simulink model "SF107A_MotRplCoggCmd"  (R2013b)
settings: Solver=FixedStepDiscrete  SolverMode=SingleTasking  StartTime=0.0  StopTime=1  FixedStep=0.002  RelTol=1e-3
undefined symbols (not defined in the file): ARCHGLBPRM_2PI_ULS_F32, ININITRNIDXCON_CNT_U16, ITRNIDXCON_CNT_U08, MotRplCoggCmdHrmncOrder1Elec, MotRplCoggCmdHrmncOrder2Elec, MotRplCoggCmdHrmncOrder3Elec, NvmGetErrSts1, ONEOVER12_MOTREV_F32, ONEOVER2PI_ULS_F32
libraries: NxtrNvM x3, NxtrLim x3, NxtrMath x3, simulink x2, FloatToFixd x2, FixdToFloat x2
(part 2 of 2)

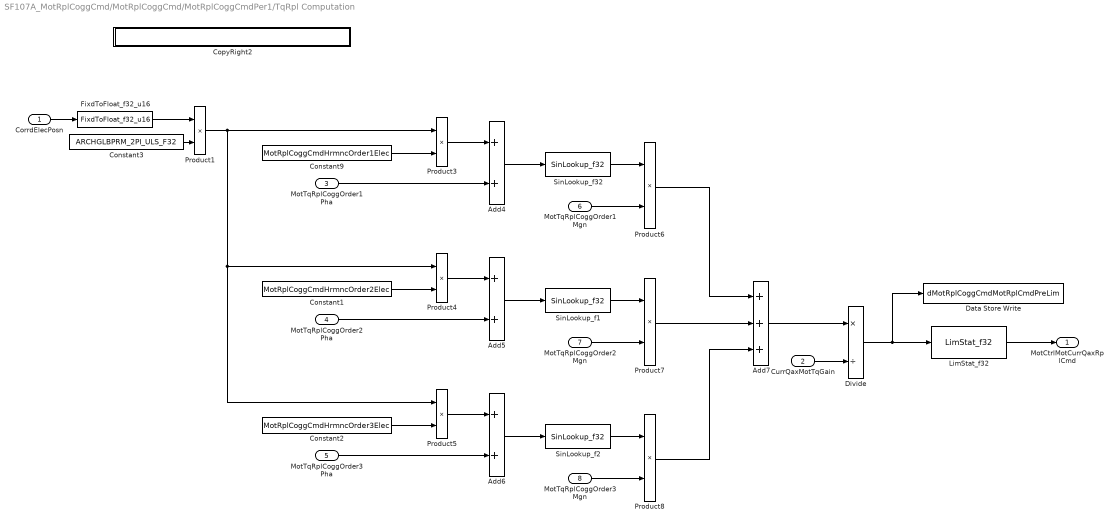
== system SF107A_MotRplCoggCmd/MotRplCoggCmd/MotRplCoggCmdPer1/TqRpl Computation ==
  CorrdElecPosn : Inport
  CurrQaxMotTqGain : Inport  Port=2
  MotTqRplCoggOrder1Pha : Inport  Port=3
  MotTqRplCoggOrder2Pha : Inport  Port=4
  MotTqRplCoggOrder3Pha : Inport  Port=5
  MotTqRplCoggOrder1Mgn : Inport  Port=6
  MotTqRplCoggOrder2Mgn : Inport  Port=7
  MotTqRplCoggOrder3Mgn : Inport  Port=8
  Add4 : Sum  RequirementInfo="{'linktype_rmi_doors' '0000bb46 (/E-STEER Core/SubSystem Specifications/Application Functions/SF99/SF107A Cogging and Ripple Command Generation)' '#SF107A_55' 'true' 'REQ:  SF107A_55' '' } %GIDa_98f659b8_5f56_4abb_a016_23e4f1dc427c"
  Add5 : Sum  RequirementInfo="{'linktype_rmi_doors' '0000bb46 (/E-STEER Core/SubSystem Specifications/Application Functions/SF99/SF107A Cogging and Ripple Command Generation)' '#SF107A_55' 'true' 'REQ:  SF107A_55' '' } %GIDa_a031d6e0_d51d_47e6_9a68_2e9a42cf15d5"
  Add6 : Sum  RequirementInfo="{'linktype_rmi_doors' '0000bb46 (/E-STEER Core/SubSystem Specifications/Application Functions/SF99/SF107A Cogging and Ripple Command Generation)' '#SF107A_55' 'true' 'REQ:  SF107A_55' '' } %GIDa_8917c88f_1d70_4c7d_a0e1_dd355f06626f"
  Add7 : Sum  RequirementInfo="{'linktype_rmi_doors' '0000bb46 (/E-STEER Core/SubSystem Specifications/Application Functions/SF99/SF107A Cogging and Ripple Command Generation)' '#SF107A_54' 'true' 'REQ:  SF107A_54' '' } %GIDa_e539927c_b2fd_444b_9336_b367779ce02b"  Inputs=+++
  Constant1 : Constant  RequirementInfo="{'linktype_rmi_doors' '0000bb46 (/E-STEER Core/SubSystem Specifications/Application Functions/SF99/SF107A Cogging and Ripple Command Generation)' '#SF107A_57' 'true' 'REQ:  SF107A_57' '' } %GIDa_f072efd8_bbd4_4d38_ae65_803309e61bdb"  Value=MotRplCoggCmdHrmncOrder2Elec
  Constant2 : Constant  RequirementInfo="{'linktype_rmi_doors' '0000bb46 (/E-STEER Core/SubSystem Specifications/Application Functions/SF99/SF107A Cogging and Ripple Command Generation)' '#SF107A_57' 'true' 'REQ:  SF107A_57' '' } %GIDa_2383bf9d_24cd_4efb_88f1_9d3d7a1f1b92"  Value=MotRplCoggCmdHrmncOrder3Elec
  Constant3 : Constant  Value=ARCHGLBPRM_2PI_ULS_F32
  Constant9 : Constant  RequirementInfo="{'linktype_rmi_doors' '0000bb46 (/E-STEER Core/SubSystem Specifications/Application Functions/SF99/SF107A Cogging and Ripple Command Generation)' '#SF107A_57' 'true' 'REQ:  SF107A_57' '' } %GIDa_68103fb0_c239_4eaa_ade4_33adb71360ab"  Value=MotRplCoggCmdHrmncOrder1Elec
  CopyRight2 : Subsystem  Description=|  mask(Copyright Information){none=on}
      | Copyright info block.                                               
      |                                                                     
      | Place copyright information at the top of every subsystem in design.
      mask prompts: none "No parameters"
      mask help: Place copyright information at the top of every subsystem in design.
      mask Display:
      | NxtrConf = 'Nexteer Confidential';
      | 
      | sys = bdroot; %handle for the current model ("system")
      | first = get_param(sys,'Created');
      | if(isempty(first))
      |     first = datestr(now,'yyyy');
      | else
      |     first = first(end-3:end);  %year is last four digits
      | end
      | 
      | last = get_param(sys,'LastModifiedDate');
      | if isempty(last)
      |     last = datestr(now,'yyyy');
      | else
      |     last = last(end-3:end);
      | end
      | 
      | if strcmp(first,last)
      |     fprintf('%s -- Copyright %s Nexteer',NxtrConf,first)
      | else
      |     fprintf('%s -- %s%s- %s Nexteer',NxtrConf,char(169),first,last)
      | end
  Data Store Write : DataStoreWrite  DataStoreName=dMotRplCoggCmdMotRplCmdPreLim
  Divide : Product  RequirementInfo="{'linktype_rmi_doors' '0000bb46 (/E-STEER Core/SubSystem Specifications/Application Functions/SF99/SF107A Cogging and Ripple Command Generation)' '#SF107A_53' 'true' 'REQ:  SF107A_53' '' } %GIDa_313ededd_ac17_4f1e_9f46_14b7bb626f21"  Inputs=*/
  FixdToFloat_f32_u16 : FixdToFloat/FixdToFloat_f32_u16  Param1=16
  LimStat_f32 : NxtrLim/LimStat_f32  LoLim=MOTRPLCMDLOLIM_AMPR_F32  HiLim=MOTRPLCMDHILIM_AMPR_F32
      settings: AttributesFormatString=|
      | Low Limit: %<LoLim>
      | High Limit:%<HiLim>
  Product1 : Product  RequirementInfo="{'linktype_rmi_doors' '0000bb46 (/E-STEER Core/SubSystem Specifications/Application Functions/SF99/SF107A Cogging and Ripple Command Generation)' '#SF107A_55' 'true' 'REQ:  SF107A_55' '' } %GIDa_600ef9ea_cc95_47b9_9c04_0003a85331d8"
  Product3 : Product  RequirementInfo="{'linktype_rmi_doors' '0000bb46 (/E-STEER Core/SubSystem Specifications/Application Functions/SF99/SF107A Cogging and Ripple Command Generation)' '#SF107A_55' 'true' 'REQ:  SF107A_55' '' } %GIDa_3469ba64_b899_493e_9d33_70a47609b0d9"
  Product4 : Product  RequirementInfo="{'linktype_rmi_doors' '0000bb46 (/E-STEER Core/SubSystem Specifications/Application Functions/SF99/SF107A Cogging and Ripple Command Generation)' '#SF107A_55' 'true' 'REQ:  SF107A_55' '' } %GIDa_836095c6_cb2f_45b0_8f00_b099e6d0c57b"
  Product5 : Product  RequirementInfo="{'linktype_rmi_doors' '0000bb46 (/E-STEER Core/SubSystem Specifications/Application Functions/SF99/SF107A Cogging and Ripple Command Generation)' '#SF107A_55' 'true' 'REQ:  SF107A_55' '' } %GIDa_688eee67_c46e_432a_b632_56124a9b3371"
  Product6 : Product  RequirementInfo="{'linktype_rmi_doors' '0000bb46 (/E-STEER Core/SubSystem Specifications/Application Functions/SF99/SF107A Cogging and Ripple Command Generation)' '#SF107A_55' 'true' 'REQ:  SF107A_55' '' } %GIDa_9339410d_3093_41b9_852e_c1514004436d"
  Product7 : Product  RequirementInfo="{'linktype_rmi_doors' '0000bb46 (/E-STEER Core/SubSystem Specifications/Application Functions/SF99/SF107A Cogging and Ripple Command Generation)' '#SF107A_55' 'true' 'REQ:  SF107A_55' '' } %GIDa_a170c4db_a53c_4e52_92bc_536d39694cf5"
  Product8 : Product  RequirementInfo="{'linktype_rmi_doors' '0000bb46 (/E-STEER Core/SubSystem Specifications/Application Functions/SF99/SF107A Cogging and Ripple Command Generation)' '#SF107A_55' 'true' 'REQ:  SF107A_55' '' } %GIDa_e07e829d_dd69_4b61_917b_3f5e8f99ba6e"
  SinLookup_f1 : NxtrMath/SinLookup_f32  RequirementInfo="{'linktype_rmi_doors' '0000bb46 (/E-STEER Core/SubSystem Specifications/Application Functions/SF99/SF107A Cogging and Ripple Command Generation)' '#SF107A_55' 'true' 'REQ:  SF107A_55' '' } %GIDa_3d2458f1_7193_4548_807d_b5b7c1c38197"
  SinLookup_f2 : NxtrMath/SinLookup_f32  RequirementInfo="{'linktype_rmi_doors' '0000bb46 (/E-STEER Core/SubSystem Specifications/Application Functions/SF99/SF107A Cogging and Ripple Command Generation)' '#SF107A_55' 'true' 'REQ:  SF107A_55' '' } %GIDa_b6162dde_f64c_4e1b_975d_22547d97ab53"
  SinLookup_f32 : NxtrMath/SinLookup_f32  RequirementInfo="{'linktype_rmi_doors' '0000bb46 (/E-STEER Core/SubSystem Specifications/Application Functions/SF99/SF107A Cogging and Ripple Command Generation)' '#SF107A_55' 'true' 'REQ:  SF107A_55' '' } %GIDa_5133dd47_8220_4bd1_8174_beaea066f0ab"
  MotCtrlMotCurrQaxRplCmd : Outport
  wires:
  Add6/1 -> SinLookup_f2/1
  Product4/1 -> Add5/1
  Product6/1 -> Add7/1
  MotTqRplCoggOrder3Mgn/1 -> Product8/2
  Constant1/1 -> Product4/2
  Product3/1 -> Add4/1
  Add4/1 -> SinLookup_f32/1
  MotTqRplCoggOrder2Mgn/1 -> Product7/2
  MotTqRplCoggOrder3Pha/1 -> Add6/2
  SinLookup_f1/1 -> Product7/1
  Add7/1 -> Divide/1
  Product8/1 -> Add7/3
  CorrdElecPosn/1 -> FixdToFloat_f32_u16/1
  Product5/1 -> Add6/1
  MotTqRplCoggOrder2Pha/1 -> Add5/2
  Constant2/1 -> Product5/2
  SinLookup_f32/1 -> Product6/1
  Product7/1 -> Add7/2
  Add5/1 -> SinLookup_f1/1
  Divide/1 -> LimStat_f32/1, Data Store Write/1
  CurrQaxMotTqGain/1 -> Divide/2
  Constant9/1 -> Product3/2
  SinLookup_f2/1 -> Product8/1
  MotTqRplCoggOrder1Pha/1 -> Add4/2
  MotTqRplCoggOrder1Mgn/1 -> Product6/2
  LimStat_f32/1 -> MotCtrlMotCurrQaxRplCmd/1
  Product1/1 -> Product4/1, Product5/1, Product3/1
  FixdToFloat_f32_u16/1 -> Product1/1
  Constant3/1 -> Product1/2

== system SF107A_MotRplCoggCmd/MotRplCoggCmd/SetMotCoggCmdPrm/CopyRight1 ==

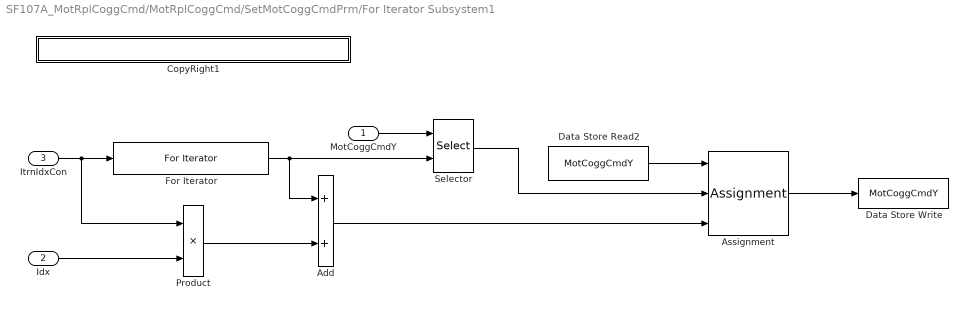
== system SF107A_MotRplCoggCmd/MotRplCoggCmd/SetMotCoggCmdPrm/For Iterator Subsystem1 ==
  MotCoggCmdY : Inport
  Idx : Inport  Port=2
  ItrnIdxCon : Inport  Port=3
  Add : Sum
  Assignment : Assignment  IndexMode=Zero-based  IndexOptions=Index vector (port)  Indices=1  OutputSizes=128
  CopyRight1 : Subsystem  Description=|  mask(Copyright Information){none=on}
      | Copyright info block.                                               
      |                                                                     
      | Place copyright information at the top of every subsystem in design.
      mask prompts: none "No parameters"
      mask help: Place copyright information at the top of every subsystem in design.
      mask Display:
      | NxtrConf = 'Nexteer Confidential';
      | 
      | sys = bdroot; %handle for the current model ("system")
      | first = get_param(sys,'Created');
      | if(isempty(first))
      |     first = datestr(now,'yyyy');
      | else
      |     first = first(end-3:end);  %year is last four digits
      | end
      | 
      | last = get_param(sys,'LastModifiedDate');
      | if isempty(last)
      |     last = datestr(now,'yyyy');
      | else
      |     last = last(end-3:end);
      | end
      | 
      | if strcmp(first,last)
      |     fprintf('%s -- Copyright %s Nexteer',NxtrConf,first)
      | else
      |     fprintf('%s -- %s%s- %s Nexteer',NxtrConf,char(169),first,last)
      | end
  Data Store Read2 : DataStoreRead  DataStoreName=MotCoggCmdY
  Data Store Write : DataStoreWrite  DataStoreName=MotCoggCmdY
  For Iterator : ForIterator  IterationSource=external  IterationLimit=127  IndexMode=Zero-based  IterationVariableDataType=int16
  Product : Product  OutDataTypeStr=int16
  Selector : Selector  IndexMode=Zero-based  InputPortWidth=128  IndexOptions=Index vector (port)  Indices=[1 3]  OutputSizes=1
  wires:
  Data Store Read2/1 -> Assignment/1
  Product/1 -> Add/2
  MotCoggCmdY/1 -> Selector/1
  Assignment/1 -> Data Store Write/1
  For Iterator/1 -> Add/1, Selector/2
  Idx/1 -> Product/2
  ItrnIdxCon/1 -> Product/1, For Iterator/1
  Add/1 -> Assignment/3
  Selector/1 -> Assignment/2

== system SF107A_MotRplCoggCmd/MotRplCoggCmd/GetMotCoggCmdPrm/For Iterator Subsystem/CopyRight1 ==

== system SF107A_MotRplCoggCmd/MotRplCoggCmd/MotRplCoggCmdInit1/NVM is NOT okay/CopyRight2 ==

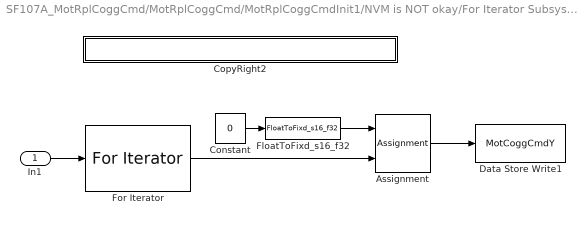
== system SF107A_MotRplCoggCmd/MotRplCoggCmd/MotRplCoggCmdInit1/NVM is NOT okay/For Iterator Subsystem ==
  In1 : Inport
  Assignment : Assignment  IndexMode=Zero-based  OutputInitialize=Specify size for each dimension in table  IndexOptions=Index vector (port)  Indices=1  OutputSizes=512
  Constant : Constant  Value=0  OutDataTypeStr=single
      settings: AttributesFormatString=%<OutDataTypeStr>
  CopyRight2 : Subsystem  Description=|  mask(Copyright Information){none=on}
      | Copyright info block.                                               
      |                                                                     
      | Place copyright information at the top of every subsystem in design.
      mask prompts: none "No parameters"
      mask help: Place copyright information at the top of every subsystem in design.
      mask Display:
      | NxtrConf = 'Nexteer Confidential';
      | 
      | sys = bdroot; %handle for the current model ("system")
      | first = get_param(sys,'Created');
      | if(isempty(first))
      |     first = datestr(now,'yyyy');
      | else
      |     first = first(end-3:end);  %year is last four digits
      | end
      | 
      | last = get_param(sys,'LastModifiedDate');
      | if isempty(last)
      |     last = datestr(now,'yyyy');
      | else
      |     last = last(end-3:end);
      | end
      | 
      | if strcmp(first,last)
      |     fprintf('%s -- Copyright %s Nexteer',NxtrConf,first)
      | else
      |     fprintf('%s -- %s%s- %s Nexteer',NxtrConf,char(169),first,last)
      | end
  Data Store Write1 : DataStoreWrite  DataStoreName=MotCoggCmdY
  FloatToFixd_s16_f32 : FloatToFixd/FloatToFixd_s16_f32  Param1=14
  For Iterator : ForIterator  IterationSource=external  IterationLimit=512  IndexMode=Zero-based  IterationVariableDataType=int16
  wires:
  In1/1 -> For Iterator/1
  For Iterator/1 -> Assignment/2
  Assignment/1 -> Data Store Write1/1
  FloatToFixd_s16_f32/1 -> Assignment/1
  Constant/1 -> FloatToFixd_s16_f32/1

== system SF107A_MotRplCoggCmd/MotRplCoggCmd/MotRplCoggCmdPer1/ Wrapping/CopyRight2 ==

== system SF107A_MotRplCoggCmd/MotRplCoggCmd/MotRplCoggCmdPer1/ Wrapping/If Action Subsystem1 ==
  Action Port : ActionPort  ActionType=then
  Constant : Constant  OutDataTypeStr=single
      settings: AttributesFormatString=%<OutDataTypeStr>
  CopyRight2 : Subsystem  Description=|  mask(Copyright Information){none=on}
      | Copyright info block.                                               
      |                                                                     
      | Place copyright information at the top of every subsystem in design.
      mask prompts: none "No parameters"
      mask help: Place copyright information at the top of every subsystem in design.
      mask Display:
      | NxtrConf = 'Nexteer Confidential';
      | 
      | sys = bdroot; %handle for the current model ("system")
      | first = get_param(sys,'Created');
      | if(isempty(first))
      |     first = datestr(now,'yyyy');
      | else
      |     first = first(end-3:end);  %year is last four digits
      | end
      | 
      | last = get_param(sys,'LastModifiedDate');
      | if isempty(last)
      |     last = datestr(now,'yyyy');
      | else
      |     last = last(end-3:end);
      | end
      | 
      | if strcmp(first,last)
      |     fprintf('%s -- Copyright %s Nexteer',NxtrConf,first)
      | else
      |     fprintf('%s -- %s%s- %s Nexteer',NxtrConf,char(169),first,last)
      | end
  Out1 : Outport
  wires:
  Constant/1 -> Out1/1

== system SF107A_MotRplCoggCmd/MotRplCoggCmd/MotRplCoggCmdPer1/ Wrapping/If Action Subsystem5 ==
  Action Port : ActionPort  ActionType=else
  Constant1 : Constant  Value=0  OutDataTypeStr=single
      settings: AttributesFormatString=%<OutDataTypeStr>
  CopyRight2 : Subsystem  Description=|  mask(Copyright Information){none=on}
      | Copyright info block.                                               
      |                                                                     
      | Place copyright information at the top of every subsystem in design.
      mask prompts: none "No parameters"
      mask help: Place copyright information at the top of every subsystem in design.
      mask Display:
      | NxtrConf = 'Nexteer Confidential';
      | 
      | sys = bdroot; %handle for the current model ("system")
      | first = get_param(sys,'Created');
      | if(isempty(first))
      |     first = datestr(now,'yyyy');
      | else
      |     first = first(end-3:end);  %year is last four digits
      | end
      | 
      | last = get_param(sys,'LastModifiedDate');
      | if isempty(last)
      |     last = datestr(now,'yyyy');
      | else
      |     last = last(end-3:end);
      | end
      | 
      | if strcmp(first,last)
      |     fprintf('%s -- Copyright %s Nexteer',NxtrConf,first)
      | else
      |     fprintf('%s -- %s%s- %s Nexteer',NxtrConf,char(169),first,last)
      | end
  Out1 : Outport
  wires:
  Constant1/1 -> Out1/1

== system SF107A_MotRplCoggCmd/MotRplCoggCmd/MotRplCoggCmdPer1/CoggTq Computation/CopyRight2 ==

== system SF107A_MotRplCoggCmd/MotRplCoggCmd/MotRplCoggCmdPer1/MotElecMeclPolarity Compensating/CopyRight2 ==

== system SF107A_MotRplCoggCmd/MotRplCoggCmd/MotRplCoggCmdPer1/MotElecMeclPolarity Compensating/Output -1//12 MotRev ==
  Action Port : ActionPort  ActionType=then
  Constant1 : Constant  Value=ONEOVER12_MOTREV_F32
  CopyRight2 : Subsystem  Description=|  mask(Copyright Information){none=on}
      | Copyright info block.                                               
      |                                                                     
      | Place copyright information at the top of every subsystem in design.
      mask prompts: none "No parameters"
      mask help: Place copyright information at the top of every subsystem in design.
      mask Display:
      | NxtrConf = 'Nexteer Confidential';
      | 
      | sys = bdroot; %handle for the current model ("system")
      | first = get_param(sys,'Created');
      | if(isempty(first))
      |     first = datestr(now,'yyyy');
      | else
      |     first = first(end-3:end);  %year is last four digits
      | end
      | 
      | last = get_param(sys,'LastModifiedDate');
      | if isempty(last)
      |     last = datestr(now,'yyyy');
      | else
      |     last = last(end-3:end);
      | end
      | 
      | if strcmp(first,last)
      |     fprintf('%s -- Copyright %s Nexteer',NxtrConf,first)
      | else
      |     fprintf('%s -- %s%s- %s Nexteer',NxtrConf,char(169),first,last)
      | end
  Unary Minus : UnaryMinus
  Out1 : Outport
  wires:
  Constant1/1 -> Unary Minus/1
  Unary Minus/1 -> Out1/1

== system SF107A_MotRplCoggCmd/MotRplCoggCmd/MotRplCoggCmdPer1/MotElecMeclPolarity Compensating/Output 1//12 MotRev ==
  Action Port : ActionPort  ActionType=else
  Constant1 : Constant  Value=ONEOVER12_MOTREV_F32
  CopyRight2 : Subsystem  Description=|  mask(Copyright Information){none=on}
      | Copyright info block.                                               
      |                                                                     
      | Place copyright information at the top of every subsystem in design.
      mask prompts: none "No parameters"
      mask help: Place copyright information at the top of every subsystem in design.
      mask Display:
      | NxtrConf = 'Nexteer Confidential';
      | 
      | sys = bdroot; %handle for the current model ("system")
      | first = get_param(sys,'Created');
      | if(isempty(first))
      |     first = datestr(now,'yyyy');
      | else
      |     first = first(end-3:end);  %year is last four digits
      | end
      | 
      | last = get_param(sys,'LastModifiedDate');
      | if isempty(last)
      |     last = datestr(now,'yyyy');
      | else
      |     last = last(end-3:end);
      | end
      | 
      | if strcmp(first,last)
      |     fprintf('%s -- Copyright %s Nexteer',NxtrConf,first)
      | else
      |     fprintf('%s -- %s%s- %s Nexteer',NxtrConf,char(169),first,last)
      | end
  Out1 : Outport
  wires:
  Constant1/1 -> Out1/1

== system SF107A_MotRplCoggCmd/MotRplCoggCmd/MotRplCoggCmdPer1/TqRpl Computation/CopyRight2 ==

== system SF107A_MotRplCoggCmd/MotRplCoggCmd/SetMotCoggCmdPrm/For Iterator Subsystem1/CopyRight1 ==

== system SF107A_MotRplCoggCmd/MotRplCoggCmd/MotRplCoggCmdInit1/NVM is NOT okay/For Iterator Subsystem/CopyRight2 ==

== system SF107A_MotRplCoggCmd/MotRplCoggCmd/MotRplCoggCmdPer1/ Wrapping/If Action Subsystem1/CopyRight2 ==

== system SF107A_MotRplCoggCmd/MotRplCoggCmd/MotRplCoggCmdPer1/ Wrapping/If Action Subsystem5/CopyRight2 ==

== system SF107A_MotRplCoggCmd/MotRplCoggCmd/MotRplCoggCmdPer1/MotElecMeclPolarity Compensating/Output -1//12 MotRev/CopyRight2 ==

== system SF107A_MotRplCoggCmd/MotRplCoggCmd/MotRplCoggCmdPer1/MotElecMeclPolarity Compensating/Output 1//12 MotRev/CopyRight2 ==
